simulink model "acc"  (R2018b)
settings: Solver=VariableStepAuto  StartTime=0.0  StopTime=20  RelTol=1e-3
values from neighbouring files (symbols this model uses):
  A = [0 1 -1; 0 0 0; 0 0 0]    [lq_controller.m]
  B = [0 0; 1 0; 0 1]    [lq_controller.m]
  C = [-1 0 t_hw; 0 e0 0]    [lq_controller.m]
  D = [0 0; 0 0]    [lq_controller.m]
  K = lqr(sys,Q,R)    [lq_controller.m]
settings Model: Creator=Nam Anh Mai The  LastModifiedBy=Nam Anh Mai The

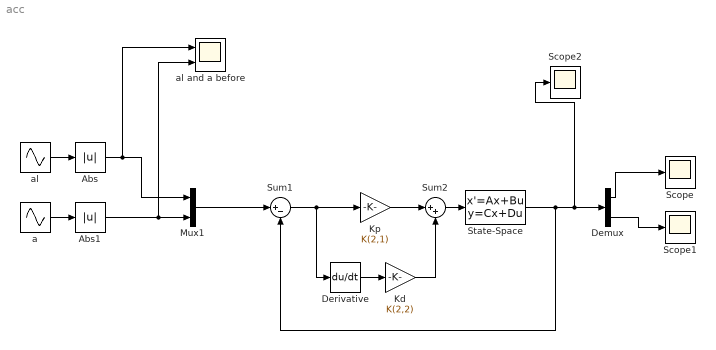
== system acc ==
  Abs : Abs
  Abs1 : Abs
  Demux : Demux  Outputs=2
  Derivative : Derivative
  "Kd " : Gain  Gain=K(2,2)
  "Kp " : Gain  Gain=K(2,1)
  Mux1 : Mux  Inputs=2
  Scope : Scope
  Scope1 : Scope
  Scope2 : Scope
  State-Space : StateSpace  A=A  B=B  C=C  D=D  InitialCondition=0
  Sum1 : Sum  Inputs=|+-
  Sum2 : Sum  Inputs=|++
  "a " : Sin  Amplitude=3  SampleTime=0.1
  al : Sin  Amplitude=4  SampleTime=0.1
  "al and a before " : Scope  NumInputPorts=2
  wires:
  Sum1/1 -> Derivative/1, "Kp "/1
  Demux/1 -> Scope/1
  Demux/2 -> Scope1/1
  "a "/1 -> Abs1/1
  al/1 -> Abs/1
  Mux1/1 -> Sum1/1
  "Kp "/1 -> Sum2/1
  State-Space/1 -> Scope2/1, Demux/1, Sum1/2
  Abs/1 -> "al and a before "/1, Mux1/1
  Abs1/1 -> "al and a before "/2, Mux1/2
  Derivative/1 -> "Kd "/1
  Sum2/1 -> State-Space/1
  "Kd "/1 -> Sum2/2
